simulink model "Simulation"  (R2023b)
settings: Solver=ode4  StartTime=0.0  StopTime=Te  FixedStep=Ts/20  RelTol=1e-3
undefined symbols (not defined in the file): EgoCar1_params, egoCarID1, targetSpeed, Ts
libraries: drivingscenarioandsensors x7, trackingutilitieslib x2, drivinglib x1, sensorinslib x1
(part 1 of 6)
settings Model: NumberOfSteps=10  SnapshotBufferSize=1000  SnapshotInterval=100  Creator=Victor  LastModifiedBy=victor
settings SolverCC: ZeroCrossAlgorithm=Adaptive
settings DebuggingCC: IgnoredZcDiagnostic=none
settings RTWCC: Toolchain=MinGW64 | CMake/gmake (64-bit Windows)  BuildConfiguration=Release

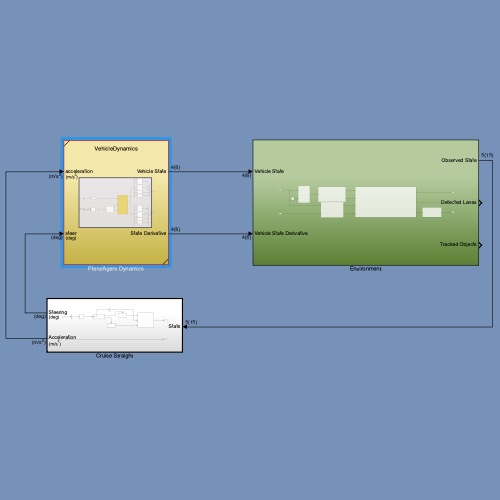
[thumbnail: Simulink's stored preview of the top-level diagram]
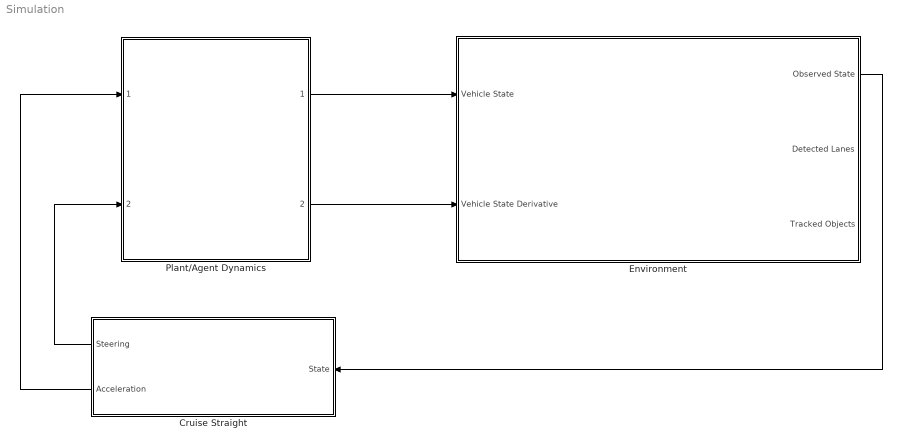
== system Simulation ==
  Cruise Straight : Subsystem  TreatAsAtomicUnit=on
  Environment : Subsystem
  Plant/Agent Dynamics : Subsystem  SystemSampleTime=Ts/20  ReferencedSubsystem=VehicleDynamics
  wires:
  Plant/Agent Dynamics/1 -> Environment/1(Vehicle State)
  Plant/Agent Dynamics/2 -> Environment/2(Vehicle State Derivative)
  Environment/1(Observed State) -> Cruise Straight/1(State)
  Cruise Straight/1(Steering) -> Plant/Agent Dynamics/2
  Cruise Straight/2(Acceleration) -> Plant/Agent Dynamics/1

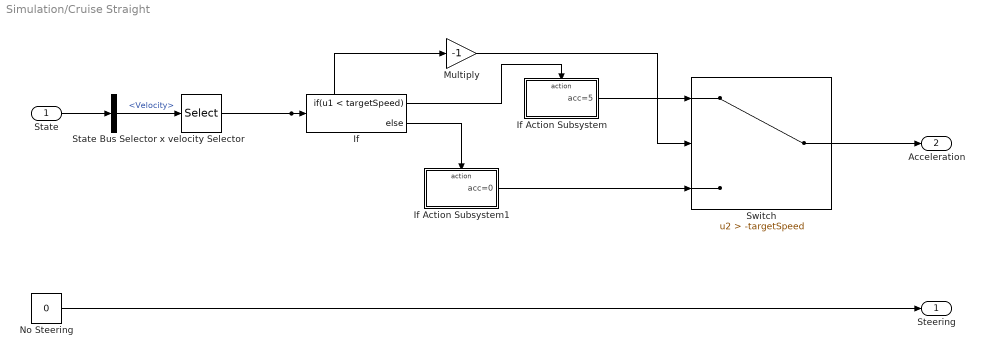
== system Simulation/Cruise Straight ==
  State : Inport
  If : If  IfExpression=u1 < targetSpeed
  If Action Subsystem : Subsystem  TreatAsAtomicUnit=on
  If Action Subsystem1 : Subsystem  TreatAsAtomicUnit=on
  Multiply : Gain  Gain=-1
  No Steering : Constant  Value=0
  State Bus Selector : BusSelector  OutputSignals=Velocity
  Switch : Switch  Criteria=u2 > Threshold  Threshold=-targetSpeed  SaturateOnIntegerOverflow=off  InputSameDT=off
  x velocity Selector : Selector  InputPortWidth=3  IndexOptions=Index vector (dialog)  Indices=[1]  OutputSizes=1
  Steering : Outport  Unit=deg
  Acceleration : Outport  Port=2  Unit=m/s^2
  wires:
  Switch/1 -> Acceleration/1
  If Action Subsystem/1(acc=5) -> Switch/1
  If/1 -> If Action Subsystem/Action
  State/1 -> State Bus Selector/1
  x velocity Selector/1 -> Multiply/1, If/1
  If Action Subsystem1/1(acc=0) -> Switch/3
  No Steering/1 -> Steering/1
  Multiply/1 -> Switch/2
  State Bus Selector/1 -> x velocity Selector/1  "<Velocity>"
  If/2 -> If Action Subsystem1/Action

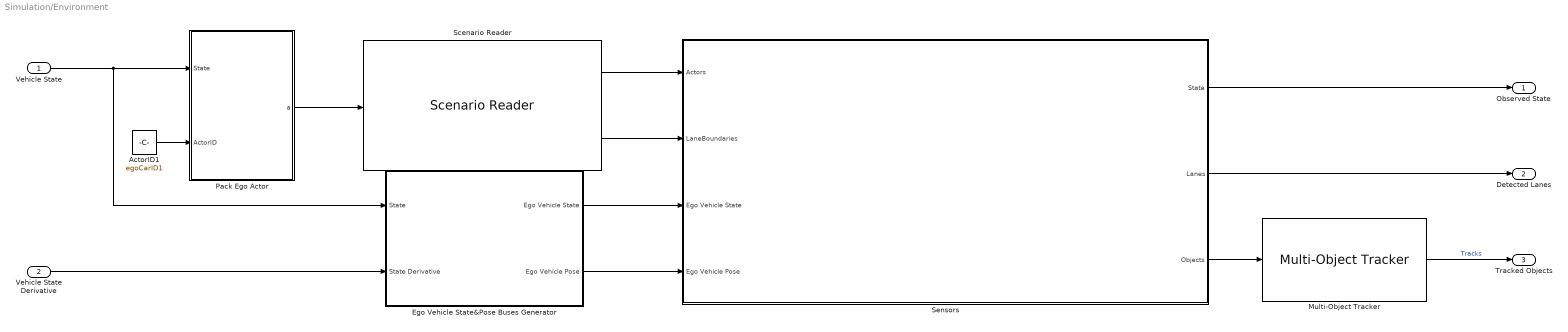
== system Simulation/Environment ==
  Vehicle State : Inport
  Vehicle State Derivative : Inport  Port=2
  ActorID1 : Constant  Value=egoCarID1
  Ego Vehicle State&Pose Buses Generator : Subsystem
  Multi-Object Tracker : drivinglib/Multi-Object Tracker  TrackerIndex=uint32( 0 )  FilterInitializationFcn=initcvekf  AssignmentThreshold=50  ConfirmationThreshold=[ 2, 3 ]  DeletionThreshold=[5,5]  MaxNumTracks=20  MaxNumSensors=8  OOSMHandling=Terminate  StateParametersSimulink=struct  HasStateParametersInput=off  TimeInputSource=Auto  HasCostMatrixInput=off  HasDetectableTrackIDsInput=off  BusNameSource=Auto  BusName=BusMultiObjectTracker1  TentativeTracksOutputPort=off  AllTracksOutputPort=off  SimulateUsing=Code generation
  Pack Ego Actor : MATLAB Function  TreatAsAtomicUnit=on
  Scenario Reader : drivingscenarioandsensors/Scenario Reader  ScenarioSource=From file  ScenarioFileName=/Users/victor/Documents/Duke/IndependentStudy/project/RNNMPC/Scenarios/StraightRoad_Challenge.mat  ScenarioVariableName=scenario  OutputCoordinateSystem=Vehicle coordinates  EgoVehicleSource=Input port  EgoVehicleActorID=1  OrientVehiclesOnRoad=on  OutputEgoVehiclePose=off  OutputEgoVehicleState=on  SampleTime=Ts  LaneBoundaryOutput=Ego vehicle lane boundaries  LaneBoundaryDistance=linspace(-15, 15, 61)  LaneBoundaryLocation=Center of lane markings  BusNameSource=Auto  BusName=BusActors  BusNumActorsSource=Scenario  BusNumActors=100  BusName2Source=Auto  BusName2=BusLaneBoundaries  BusNumLaneBoundariesSource=Scenario  BusNumLaneBoundaries=10  BusName3Source=Auto  BusName3=BusEgoActor  BusName4Source=Auto  BusName4=BusEgoState  ShowCoordinateLabels=on  SimulateUsing=Code generation
  Sensors : Subsystem
  Observed State : Outport
  Detected Lanes : Outport  Port=2
  Tracked Objects : Outport  Port=3
  wires:
  Ego Vehicle State&Pose Buses Generator/2(Ego Vehicle Pose) -> Sensors/4(Ego Vehicle Pose)
  Pack Ego Actor/1(a) -> Scenario Reader/1
  Ego Vehicle State&Pose Buses Generator/1(Ego Vehicle State) -> Sensors/3(Ego Vehicle State)
  ActorID1/1 -> Pack Ego Actor/2(ActorID)
  Scenario Reader/1 -> Sensors/1(Actors)
  Vehicle State/1 -> Ego Vehicle State&Pose Buses Generator/1(State), Pack Ego Actor/1(State)
  Scenario Reader/2 -> Sensors/2(LaneBoundaries)
  Vehicle State Derivative/1 -> Ego Vehicle State&Pose Buses Generator/2(State Derivative)
  Sensors/1(State) -> Observed State/1
  Sensors/2(Lanes) -> Detected Lanes/1
  Sensors/3(Objects) -> Multi-Object Tracker/1
  Multi-Object Tracker/1 -> Tracked Objects/1  "Tracks"

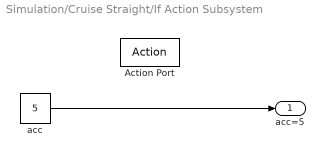
== system Simulation/Cruise Straight/If Action Subsystem ==
  Action Port : ActionPort  ActionPortLabel=if(u1 < targetSpeed)
  acc : Constant  Value=5
  acc=5 : Outport
  wires:
  acc/1 -> acc=5/1

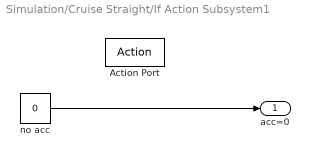
== system Simulation/Cruise Straight/If Action Subsystem1 ==
  Action Port : ActionPort  ActionPortLabel=else
  no acc : Constant  Value=0
  acc=0 : Outport
  wires:
  no acc/1 -> acc=0/1

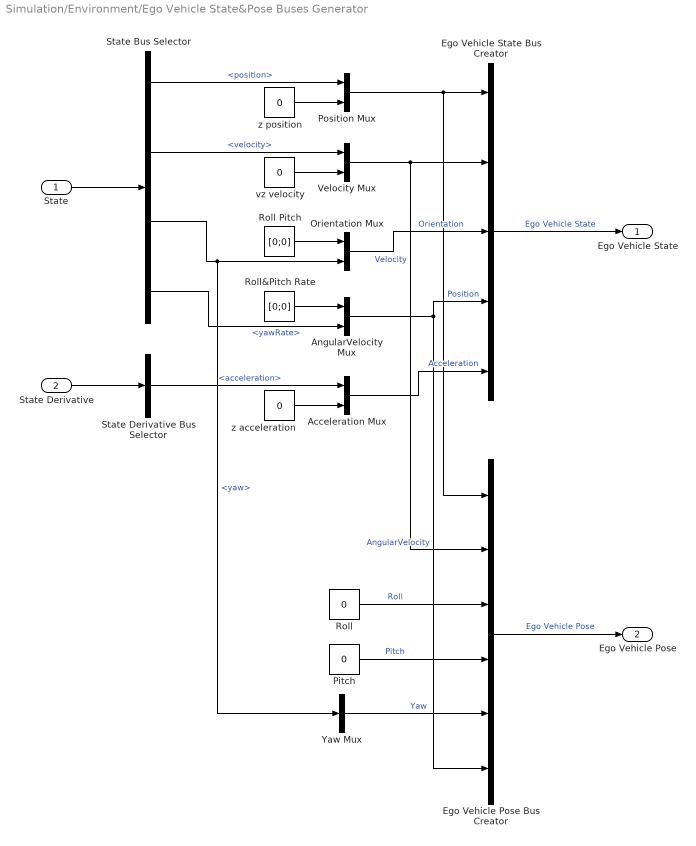
== system Simulation/Environment/Ego Vehicle State&Pose Buses Generator ==
  State : Inport
  State Derivative : Inport  Port=2
  Acceleration Mux : Mux  Inputs=2
  AngularVelocity Mux : Mux  Inputs=2
  Ego Vehicle Pose Bus Creator : BusCreator  Inputs=6
  Ego Vehicle State Bus Creator : BusCreator  Inputs=5
  Orientation Mux : Mux  Inputs=2
  Pitch : Constant  Value=0
  Position Mux : Mux  Inputs=2
  Roll : Constant  Value=0
  Roll Pitch : Constant  Value=[0;0]
  Roll&Pitch Rate : Constant  Value=[0;0]
  State Bus Selector : BusSelector  OutputSignals=position,velocity,yaw,yawRate
  State Derivative Bus Selector : BusSelector  OutputSignals=acceleration
  Velocity Mux : Mux  Inputs=2
  Yaw Mux : Mux  Inputs=1
  vz velocity : Constant  Value=0
  z acceleration : Constant  Value=0
  z position : Constant  Value=0
  Ego Vehicle State : Outport
  Ego Vehicle Pose : Outport  Port=2
  wires:
  State Derivative/1 -> State Derivative Bus Selector/1
  State Bus Selector/3 -> Orientation Mux/2, Yaw Mux/1  "<yaw>"
  Ego Vehicle State Bus Creator/1 -> Ego Vehicle State/1  "Ego Vehicle State"
  z acceleration/1 -> Acceleration Mux/2
  State Bus Selector/2 -> Velocity Mux/1  "<velocity>"
  State Bus Selector/1 -> Position Mux/1  "<position>"
  State Derivative Bus Selector/1 -> Acceleration Mux/1  "<acceleration>"
  Roll&Pitch Rate/1 -> AngularVelocity Mux/1
  z position/1 -> Position Mux/2
  vz velocity/1 -> Velocity Mux/2
  Roll Pitch/1 -> Orientation Mux/1
  Orientation Mux/1 -> Ego Vehicle State Bus Creator/3  "Orientation"
  AngularVelocity Mux/1 -> Ego Vehicle Pose Bus Creator/6, Ego Vehicle State Bus Creator/4  "AngularVelocity"
  Velocity Mux/1 -> Ego Vehicle Pose Bus Creator/2, Ego Vehicle State Bus Creator/2  "Velocity"
  State/1 -> State Bus Selector/1
  Position Mux/1 -> Ego Vehicle Pose Bus Creator/1, Ego Vehicle State Bus Creator/1  "Position"
  Acceleration Mux/1 -> Ego Vehicle State Bus Creator/5  "Acceleration"
  State Bus Selector/4 -> AngularVelocity Mux/2  "<yawRate>"
  Roll/1 -> Ego Vehicle Pose Bus Creator/3  "Roll"
  Pitch/1 -> Ego Vehicle Pose Bus Creator/4  "Pitch"
  Yaw Mux/1 -> Ego Vehicle Pose Bus Creator/5  "Yaw"
  Ego Vehicle Pose Bus Creator/1 -> Ego Vehicle Pose/1  "Ego Vehicle Pose"
